simulink model "Cuantificador3"  (R2013a)
settings: Solver=ode45  StartTime=0.0  StopTime=3.7874  RelTol=1e-3
undefined symbols (not defined in the file or in its folder): sgn
settings Model: Creator=Alfonso  LastModifiedBy=Alfonso

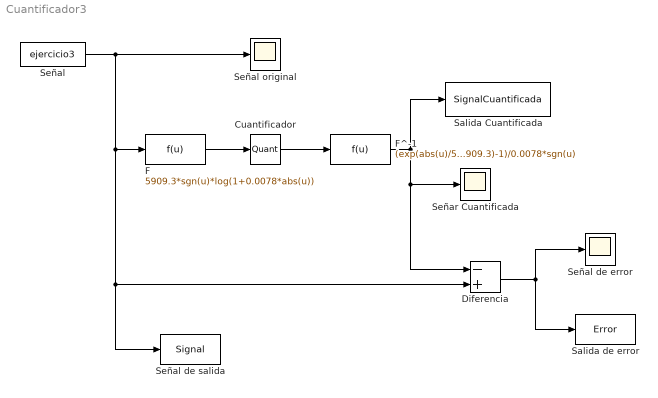
== system Cuantificador3 ==
  Cuantificador : Quantizer  QuantizationInterval=256
  Diferencia : Sum  Inputs=-+
  F : Fcn  Expr=5909.3*sgn(u)*log(1+0.0078*abs(u))
  F^-1 : Fcn  Expr=(exp(abs(u)/5909.3)-1)/0.0078*sgn(u)
  Salida Cuantificada : ToWorkspace  VariableName=SignalCuantificada  SampleTime=-1
  Salida de error : ToWorkspace  VariableName=Error  SampleTime=-1
  Señal : FromWorkspace  VariableName=ejercicio3  SampleTime=1/8000
  Señal de error : Scope
      settings: YMin=-150  YMax=150
  Señal de salida : ToWorkspace  VariableName=Signal  SampleTime=-1
  Señal original : Scope
      settings: YMin=-10000  YMax=15000  SaveName=ScopeData2
  Señar Cuantificada : Scope
      settings: YMin=-10000  YMax=15000
  wires:
  Señal/1 -> F/1, Diferencia/2, Señal de salida/1, Señal original/1
  Diferencia/1 -> Salida de error/1, Señal de error/1
  F/1 -> Cuantificador/1
  Cuantificador/1 -> F^-1/1
  F^-1/1 -> Diferencia/1, Señar Cuantificada/1, Salida Cuantificada/1
